simulink model "pn_dopple"  (Simulink 7.2)
settings: Solver=ode45  StartTime=0.0  StopTime=0.02  RelTol=1e-3
libraries: simulink x256, commsynccomp2 x2, dsparch4 x1, commfilt2 x1, commutil2 x1, dspspect3 x1
(part 1 of 3)
settings Model: Creator=Administrator  LastModifiedBy=Administrator
settings OptimizationCC: InitFltsAndDblsToZero=on

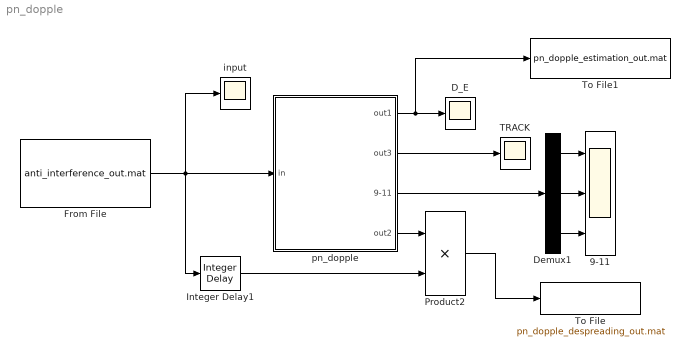
== system pn_dopple ==
  9-11 : Scope  NumInputPorts=3
      settings: YMin=0~0~0  YMax=35~35~40  SaveName=ScopeData3
  D_E : Scope
      settings: TimeRange=0.02  YMin=95  YMax=105  SaveName=ScopeData7
  Demux1 : Demux  Outputs=3
  From File : FromFile  FileName=anti_interference_out.mat  SampleTime=0
  Integer Delay1 : simulink/Discrete/Integer Delay  vinit=0.0  samptime=1/5.1e6  NumDelays=50
  Product2 : Product  OutDataType=sfix(16)  OutScaling=2^0  RndMeth=Zero
  TRACK : Scope
      settings: YMin=-1  YMax=1  SaveName=ScopeData6
  To File : ToFile  Filename=pn_dopple_despreading_out.mat  SampleTime=1/5.1e6
  To File1 : ToFile  Filename=pn_dopple_estimation_out.mat  SampleTime=1/5.1e6
  input : Scope
      settings: YMin=-1  YMax=1  SaveName=ScopeData14
  pn_dopple : Subsystem  TreatAsAtomicUnit=on
  wires:
  pn_dopple/1(out1) -> D_E/1, To File1/1
  pn_dopple/2(out3) -> TRACK/1
  pn_dopple/3(9-11) -> Demux1/1
  Demux1/1 -> 9-11/1
  Demux1/2 -> 9-11/2
  Demux1/3 -> 9-11/3
  From File/1 -> pn_dopple/1(in), Integer Delay1/1, input/1
  pn_dopple/4(out2) -> Product2/1
  Integer Delay1/1 -> Product2/2
  Product2/1 -> To File/1

== system pn_dopple/pn_dopple ==
  in : Inport  OutDataType=sfix(16)  OutScaling=2^0
  "De-Carrier " : Subsystem
  FFT compensate : Subsystem
  Local PN : Subsystem
  MF_Sstem : Subsystem
  Magnitude FFT : dspspect3/Magnitude FFT  SystemSampleTime=-1  mag_or_magsq=Magnitude  fftLenInherit=off  fftsize=32
  MainTain System : Subsystem  TreatAsAtomicUnit=on
  Scope2 : Scope
      settings: TimeRange=0.06427185951473757  YMin=-2  YMax=2  MaxDataPoints=100000
  Sign : Signum
  Zero-Order Hold : ZeroOrderHold  SampleTime=1/255e3
  out1 : Outport  OutDataType=sfix(16)  OutScaling=2^0
  out3 : Outport  Port=2  OutDataType=sfix(16)  OutScaling=2^0
  9-11 : Outport  Port=3  OutDataType=sfix(16)  OutScaling=2^0
  out2 : Outport  Port=4  OutDataType=sfix(16)  OutScaling=2^0
  wires:
  in/1 -> "De-Carrier "/1(in)
  FFT compensate/2(PN Peak) -> Local PN/1(in)
  Zero-Order Hold/1 -> Sign/1
  Sign/1 -> MF_Sstem/1(In1), Local PN/2(in1)
  MF_Sstem/1(bus Out1) -> Magnitude FFT/1
  Magnitude FFT/1 -> FFT compensate/1(In1)
  MainTain System/1(Out1) -> out1/1, Scope2/1
  "De-Carrier "/1(out) -> Zero-Order Hold/1
  Local PN/2(out) -> out3/1
  FFT compensate/3(9-11) -> 9-11/1
  FFT compensate/1(FFT compensate positive) -> MainTain System/Trigger, MainTain System/1(In1)
  Local PN/1(1 0 0 1 1 1 0 1) -> out2/1

== system pn_dopple/pn_dopple/De-Carrier  ==
  note: 5.1e5 Hz
      |
      | 1/5.1e6
      |
      | 255K-300K
  in : Inport  OutDataType=sfix(16)  OutScaling=2^0
  Continuous-Time VCO1 : commsynccomp2/Continuous-Time VCO  SystemSampleTime=-1  Ac=1  Fc=5.0e5  Kc=1000  Ph=pi/2
  Digital Filter Design4 : dsparch4/Digital Filter Design  SystemSampleTime=-1  mwdsp_browser_bugfix_var=off
  Product1 : Product  OutDataType=sfix(16)  OutScaling=2^0  RndMeth=Zero
  Scope1 : Scope
      settings: SaveName=ScopeData4  MaxDataPoints=100000
  Scope3 : Scope
      settings: SaveName=ScopeData16  MaxDataPoints=100000
  Zero-Order Hold1 : ZeroOrderHold  SampleTime=1/5.1e6
  Zero-Order Hold2 : ZeroOrderHold  SampleTime=1/5.1e6
  out : Outport  OutDataType=sfix(16)  OutScaling=2^0
  wires:
  in/1 -> Product1/2
  Product1/1 -> Scope3/1, Zero-Order Hold1/1
  Digital Filter Design4/1 -> out/1, Scope1/1
  Continuous-Time VCO1/1 -> Zero-Order Hold2/1
  Zero-Order Hold2/1 -> Product1/1
  Zero-Order Hold1/1 -> Digital Filter Design4/1

== system pn_dopple/pn_dopple/FFT compensate ==
  In1 : Inport  OutDataType=sfix(16)  OutScaling=2^0
  Demux : Demux  Outputs=32
  Mux : Mux  Inputs=3
  Product1 : Product  OutDataType=sfix(16)  OutScaling=2^0  RndMeth=Zero
  Product8 : Product  OutDataType=sfix(16)  OutScaling=2^0  RndMeth=Zero
  Rate Transition1 : RateTransition  Deterministic=off  OutPortSampleTime=1/5.1e6
  Rate Transition2 : RateTransition  Deterministic=off  OutPortSampleTime=1/5.1e6
  Rate Transition3 : RateTransition  Deterministic=off  OutPortSampleTime=1/5.1e6
  Scope{1..2,4..7} (6 alike) : Scope  NumInputPorts=3
      Scope1 settings: TimeRange=0.06427185951473757  YMin=0~-5~-5  YMax=14~5~5  SaveName=ScopeData9  MaxDataPoints=100000
      Scope2 settings: TimeRange=0.06427185951473757  YMin=0~-5~-5  YMax=14~5~5  SaveName=ScopeData11  MaxDataPoints=100000
      Scope4 settings: TimeRange=0.06427185951473757  YMin=0~-5~-5  YMax=14~5~5  SaveName=ScopeData12  MaxDataPoints=100000
      Scope5 settings: TimeRange=0.06427185951473757  YMin=0~-5~-5  YMax=14~5~5  SaveName=ScopeData13  MaxDataPoints=100000
      Scope6 settings: TimeRange=0.06427185951473757  YMin=0~-5~-5  YMax=14~5~5  SaveName=ScopeData33  MaxDataPoints=100000
      Scope7 settings: TimeRange=0.06427185951473757  YMin=0~-5~-5  YMax=14~5~5  SaveName=ScopeData47  MaxDataPoints=100000
  Scope14 : Scope
      settings: SaveName=ScopeData24  MaxDataPoints=100000
  Scope3 : Scope
      settings: SaveName=ScopeData27  MaxDataPoints=100000
  Step : Step  Time=0.001  SampleTime=0
  Step1 : Step  Time=0.001  SampleTime=0
  Subsystem : Subsystem
  FFT compensate positive : Outport  OutDataType=sfix(16)  OutScaling=2^0
  PN Peak : Outport  Port=2  OutDataType=sfix(16)  OutScaling=2^0
  9-11 : Outport  Port=3  OutDataType=sfix(16)  OutScaling=2^0
  wires:
  Demux/3 -> Subsystem/3(In3), Scope2/3
  Demux/2 -> Subsystem/2(In2), Scope2/2
  Demux/4 -> Scope1/1, Subsystem/4(In4)
  Demux/5 -> Scope1/2, Subsystem/5(In5)
  Demux/6 -> Scope1/3, Subsystem/6(In6)
  Demux/7 -> Subsystem/7(In7), Scope4/1
  Demux/8 -> Subsystem/8(In8), Scope4/2
  Demux/9 -> Subsystem/9(In9), Scope4/3
  Demux/10 -> Subsystem/10(In10), Scope5/1, Mux/1
  Demux/11 -> Subsystem/11(In11), Scope5/2, Mux/2
  Demux/12 -> Subsystem/12(In12), Scope5/3, Mux/3
  Demux/13 -> Subsystem/13(In13), Scope6/1
  Demux/14 -> Subsystem/14(In14), Scope6/2
  Demux/15 -> Subsystem/15(In15), Scope6/3
  In1/1 -> Demux/1
  Demux/1 -> Subsystem/1(In1), Scope2/1
  Subsystem/1(Out1) -> Scope14/1, Product1/1
  Step/1 -> Rate Transition3/1
  Product8/1 -> Rate Transition1/1
  Subsystem/2(Out2) -> Rate Transition2/1
  Rate Transition1/1 -> PN Peak/1, Scope3/1
  Rate Transition2/1 -> Product8/1
  Demux/16 -> Subsystem/16(In16), Scope7/1
  Demux/17 -> Scope7/2
  Demux/18 -> Scope7/3
  Rate Transition3/1 -> Product8/2
  Step1/1 -> Product1/2
  Product1/1 -> FFT compensate positive/1
  Mux/1 -> 9-11/1

== system pn_dopple/pn_dopple/Local PN ==
  in : Inport  OutDataType=sfix(16)  OutScaling=2^0
  in1 : Inport  Port=2  OutDataType=sfix(16)  OutScaling=2^0
  LOCAL_DELAY : Subsystem  TreatAsAtomicUnit=on
  PN_TRACK : Subsystem  TreatAsAtomicUnit=on
  Scope{1..5} (5 alike) : Scope
      Scope1 settings: TimeRange=0.06427185951473757  YMin=-2  YMax=2  SaveName=ScopeData23  MaxDataPoints=100000
      Scope2 settings: TimeRange=0.06427185951473757  YMin=-2  YMax=2  SaveName=ScopeData29  MaxDataPoints=100000
      Scope3 settings: TimeRange=0.06427185951473757  YMin=-2  YMax=2  SaveName=ScopeData18  MaxDataPoints=100000
      Scope4 settings: TimeRange=0.06427185951473757  YMin=-2  YMax=2  SaveName=ScopeData5  MaxDataPoints=100000
      Scope5 settings: TimeRange=0.06427185951473757  YMin=-2  YMax=2  SaveName=ScopeData30  MaxDataPoints=100000
  "local PN " : Subsystem  TreatAsAtomicUnit=on
  logic control : Subsystem  TreatAsAtomicUnit=on
  threshold deside : Subsystem  TreatAsAtomicUnit=on
  threshold deside stop and start : Subsystem
  1 0 0 1 1 1 0 1 : Outport  OutDataType=sfix(16)  OutScaling=2^0
  out : Outport  Port=2  OutDataType=sfix(16)  OutScaling=2^0
  wires:
  logic control/1(Out2) -> Scope5/1, "local PN "/Enable, PN_TRACK/Enable
  threshold deside/1(Out2) -> logic control/1(In1), threshold deside stop and start/1(In1)
  threshold deside stop and start/1(Out1) -> Scope3/1, threshold deside/Enable, Scope4/1
  [A] -> threshold deside stop and start/2(In2)
  in/1 -> threshold deside/1(In1), Scope2/1
  "local PN "/1("1 0 0 1 1 1 0 1 ") -> 1 0 0 1 1 1 0 1/1, Scope1/1, PN_TRACK/1(In1)
  PN_TRACK/1(Out1) -> "local PN "/1(B), out/1
  in1/1 -> LOCAL_DELAY/1(In1)
  LOCAL_DELAY/2(Out1) -> PN_TRACK/3(In3)
  LOCAL_DELAY/1(Out2) -> PN_TRACK/2(In2)

== system pn_dopple/pn_dopple/MF_Sstem ==
  In1 : Inport  OutDataType=sfix(16)  OutScaling=2^0
  Add : Sum  Inputs=++++++++++++++++++++++++++++++++  OutDataType=sfix(16)  OutScaling=2^-10
  MF array : Subsystem
  Mux : Mux  Inputs=32
  Scope14 : Scope
      settings: SaveName=ScopeData34  MaxDataPoints=100000
  Zero-Order Hold : ZeroOrderHold  SampleTime=1/255000
  bus Out1 : Outport  OutDataType=sfix(16)  OutScaling=2^0
  wires:
  In1/1 -> Zero-Order Hold/1
  Zero-Order Hold/1 -> MF array/1(In1)
  Mux/1 -> bus Out1/1
  Add/1 -> Scope14/1
  MF array/1(Out1) -> Mux/1, Add/1
  MF array/2(Out2) -> Mux/2, Add/2
  MF array/3(Out3) -> Mux/3, Add/3
  MF array/4(Out4) -> Mux/4, Add/4
  MF array/5(Out5) -> Mux/5, Add/5
  MF array/6(Out6) -> Mux/6, Add/6
  MF array/7(Out7) -> Mux/7, Add/7
  MF array/8(Out8) -> Mux/8, Add/8
  MF array/9(Out9) -> Mux/9, Add/9
  MF array/10(Out10) -> Mux/10, Add/10
  MF array/11(Out11) -> Mux/11, Add/11
  MF array/12(Out12) -> Mux/12, Add/12
  MF array/13(Out13) -> Mux/13, Add/13
  MF array/14(Out14) -> Mux/14, Add/14
  MF array/15(Out15) -> Mux/15, Add/15
  MF array/16(Out16) -> Mux/16, Add/16
  MF array/17(Out17) -> Mux/17, Add/17
  MF array/18(Out18) -> Mux/18, Add/18
  MF array/19(Out19) -> Mux/19, Add/19
  MF array/20(Out20) -> Mux/20, Add/20
  MF array/21(Out21) -> Mux/21, Add/21
  MF array/22(Out22) -> Mux/22, Add/22
  MF array/23(Out23) -> Mux/23, Add/23
  MF array/24(Out24) -> Mux/24, Add/24
  MF array/25(Out25) -> Mux/25, Add/25
  MF array/26(Out26) -> Mux/26, Add/26
  MF array/27(Out27) -> Mux/27, Add/27
  MF array/28(Out28) -> Mux/28, Add/28
  MF array/29(Out29) -> Mux/29, Add/29
  MF array/30(Out30) -> Mux/30, Add/30
  MF array/31(Out31) -> Mux/31, Add/31
  MF array/32(Out32) -> Mux/32, Add/32

== system pn_dopple/pn_dopple/MainTain System ==
  In1 : Inport  OutDataType=sfix(16)  OutScaling=2^0
  Trigger : TriggerPort
  Out1 : Outport  OutDataType=sfix(16)  OutScaling=2^0
  wires:
  In1/1 -> Out1/1

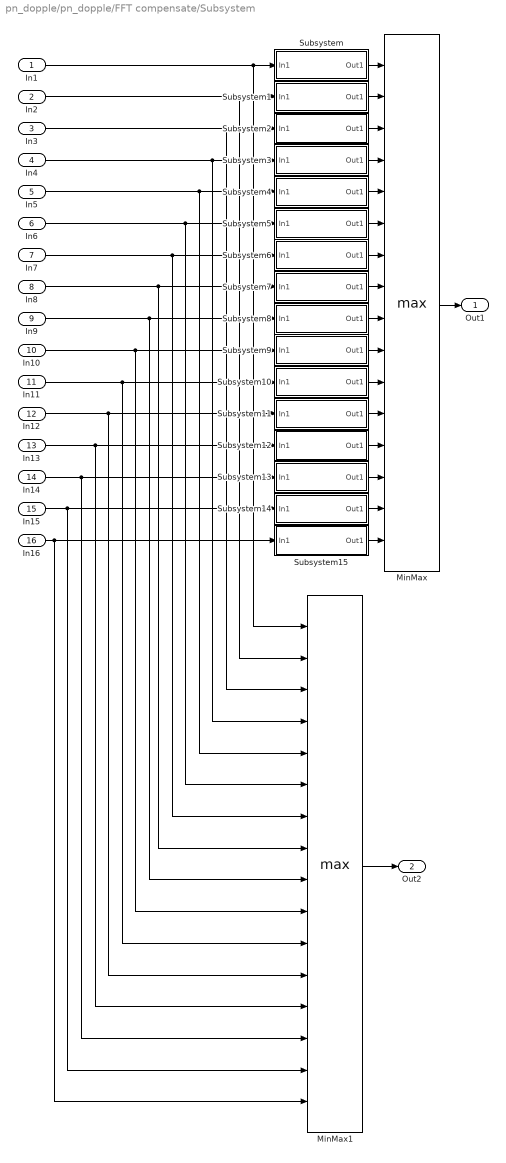
== system pn_dopple/pn_dopple/FFT compensate/Subsystem ==
  In1 : Inport  OutDataType=sfix(16)  OutScaling=2^0
  In2 : Inport  Port=2  OutDataType=sfix(16)  OutScaling=2^0
  In3 : Inport  Port=3  OutDataType=sfix(16)  OutScaling=2^0
  In4 : Inport  Port=4  OutDataType=sfix(16)  OutScaling=2^0
  In5 : Inport  Port=5  OutDataType=sfix(16)  OutScaling=2^0
  In6 : Inport  Port=6  OutDataType=sfix(16)  OutScaling=2^0
  In7 : Inport  Port=7  OutDataType=sfix(16)  OutScaling=2^0
  In8 : Inport  Port=8  OutDataType=sfix(16)  OutScaling=2^0
  In9 : Inport  Port=9  OutDataType=sfix(16)  OutScaling=2^0
  In10 : Inport  Port=10  OutDataType=sfix(16)  OutScaling=2^0
  In11 : Inport  Port=11  OutDataType=sfix(16)  OutScaling=2^0
  In12 : Inport  Port=12  OutDataType=sfix(16)  OutScaling=2^0
  In13 : Inport  Port=13  OutDataType=sfix(16)  OutScaling=2^0
  In14 : Inport  Port=14  OutDataType=sfix(16)  OutScaling=2^0
  In15 : Inport  Port=15  OutDataType=sfix(16)  OutScaling=2^0
  In16 : Inport  Port=16  OutDataType=sfix(16)  OutScaling=2^0
  MinMax : MinMax  Function=max  Inputs=16  OutDataType=sfix(16)  OutScaling=2^0
  MinMax1 : MinMax  Function=max  Inputs=16  OutDataType=sfix(16)  OutScaling=2^0
  Subsystem : Subsystem
  Subsystem1 : Subsystem
  Subsystem10 : Subsystem
  Subsystem11 : Subsystem
  Subsystem12 : Subsystem
  Subsystem13 : Subsystem
  Subsystem14 : Subsystem
  Subsystem15 : Subsystem
  Subsystem2 : Subsystem
  Subsystem3 : Subsystem
  Subsystem4 : Subsystem
  Subsystem5 : Subsystem
  Subsystem6 : Subsystem
  Subsystem7 : Subsystem
  Subsystem8 : Subsystem
  Subsystem9 : Subsystem
  Out1 : Outport  OutDataType=sfix(16)  OutScaling=2^0
  Out2 : Outport  Port=2  OutDataType=sfix(16)  OutScaling=2^0
  wires:
  In1/1 -> Subsystem/1(In1), MinMax1/1
  In2/1 -> Subsystem1/1(In1), MinMax1/2
  In3/1 -> Subsystem2/1(In1), MinMax1/3
  In4/1 -> Subsystem3/1(In1), MinMax1/4
  In5/1 -> Subsystem4/1(In1), MinMax1/5
  In6/1 -> Subsystem5/1(In1), MinMax1/6
  In7/1 -> Subsystem6/1(In1), MinMax1/7
  In8/1 -> Subsystem7/1(In1), MinMax1/8
  In9/1 -> Subsystem8/1(In1), MinMax1/9
  In10/1 -> Subsystem9/1(In1), MinMax1/10
  In11/1 -> Subsystem10/1(In1), MinMax1/11
  In12/1 -> Subsystem11/1(In1), MinMax1/12
  In13/1 -> Subsystem12/1(In1), MinMax1/13
  In14/1 -> Subsystem13/1(In1), MinMax1/14
  In15/1 -> Subsystem14/1(In1), MinMax1/15
  In16/1 -> Subsystem15/1(In1), MinMax1/16
  MinMax/1 -> Out1/1
  Subsystem/1(Out1) -> MinMax/1
  Subsystem1/1(Out1) -> MinMax/2
  Subsystem2/1(Out1) -> MinMax/3
  Subsystem3/1(Out1) -> MinMax/4
  Subsystem4/1(Out1) -> MinMax/5
  Subsystem5/1(Out1) -> MinMax/6
  Subsystem6/1(Out1) -> MinMax/7
  Subsystem7/1(Out1) -> MinMax/8
  Subsystem8/1(Out1) -> MinMax/9
  Subsystem9/1(Out1) -> MinMax/10
  Subsystem10/1(Out1) -> MinMax/11
  Subsystem11/1(Out1) -> MinMax/12
  Subsystem12/1(Out1) -> MinMax/13
  Subsystem13/1(Out1) -> MinMax/14
  Subsystem14/1(Out1) -> MinMax/15
  Subsystem15/1(Out1) -> MinMax/16
  MinMax1/1 -> Out2/1

== system pn_dopple/pn_dopple/Local PN/LOCAL_DELAY ==
  In1 : Inport  OutDataType=sfix(16)  OutScaling=2^0
  Unit Delay : UnitDelay  SampleTime=1/1000000
  Out2 : Outport  OutDataType=sfix(16)  OutScaling=2^0
  Out1 : Outport  Port=2  OutDataType=sfix(16)  OutScaling=2^0
  wires:
  In1/1 -> Unit Delay/1, Out1/1
  Unit Delay/1 -> Out2/1

== system pn_dopple/pn_dopple/Local PN/PN_TRACK ==
  In1 : Inport  OutDataType=sfix(16)  OutScaling=2^0
  In2 : Inport  Port=2  OutDataType=sfix(16)  OutScaling=2^0
  In3 : Inport  Port=3  OutDataType=sfix(16)  OutScaling=2^0
  Enable : EnablePort
  Data Type Conversion : DataTypeConversion  OutDataTypeMode=double  OutDataType=sfix(16)  OutScaling=2^0  OutDataTypeStr=double
  Data Type Conversion1 : DataTypeConversion  OutDataTypeMode=double  OutDataType=sfix(16)  OutScaling=2^0  OutDataTypeStr=double
  Data Type Conversion2 : DataTypeConversion  OutDataTypeMode=double  OutDataType=sfix(16)  OutScaling=2^0  OutDataTypeStr=double
  Gain1 : Gain  Gain=1100/1000  ParameterDataType=sfix(16)  ParameterScaling=2^0  OutDataType=sfix(16)  OutScaling=2^0
  Integrate and Dump : Subsystem
  Memory1 : Memory
  Memory2 : Memory
  Memory3 : Memory
  Product : Product  OutDataType=sfix(16)  OutScaling=2^0  RndMeth=Zero
  Product1 : Product  OutDataType=sfix(16)  OutScaling=2^0  RndMeth=Zero
  Scope : Scope  NumInputPorts=2
      settings: YMin=-5~-5  YMax=5~5  SaveName=ScopeData8
  Sum : Sum  Inputs=-+  OutDataType=sfix(16)  OutScaling=2^0
  Zero-Order Hold : ZeroOrderHold  SampleTime=10
  Zero-Order Hold1 : ZeroOrderHold  SampleTime=10
  Zero-Order Hold2 : ZeroOrderHold  SampleTime=10
  Zero-Order Hold3 : ZeroOrderHold
  Out1 : Outport  OutDataType=sfix(16)  OutScaling=2^0
  wires:
  In1/1 -> Memory1/1
  In2/1 -> Memory2/1
  In3/1 -> Memory3/1
  Data Type Conversion/1 -> Zero-Order Hold/1
  Data Type Conversion1/1 -> Zero-Order Hold1/1
  Data Type Conversion2/1 -> Zero-Order Hold2/1
  Zero-Order Hold/1 -> Product/1, Product1/1
  Zero-Order Hold1/1 -> Product/2
  Zero-Order Hold2/1 -> Product1/2
  Product/1 -> Sum/1, Scope/1
  Product1/1 -> Sum/2, Scope/2
  Sum/1 -> Zero-Order Hold3/1
  Zero-Order Hold3/1 -> Integrate and Dump/1(In1)
  Integrate and Dump/1(Out1) -> Gain1/1
  Memory1/1 -> Data Type Conversion/1
  Memory2/1 -> Data Type Conversion1/1
  Memory3/1 -> Data Type Conversion2/1
  Gain1/1 -> Out1/1

== system pn_dopple/pn_dopple/Local PN/local PN  ==
  B : Inport  OutDataType=sfix(16)  OutScaling=2^0
  Enable : EnablePort  StatesWhenEnabling=reset
  Clock : Subsystem
  Local System : Subsystem
  Scope1 : Scope
      settings: YMin=0.95  YMax=1.05  SaveName=ScopeData10
  Scope2 : Scope
      settings: YMin=0.95  YMax=1.05  SaveName=ScopeData26
  Unipolar to Bipolar Converter : commutil2/Unipolar to Bipolar Converter  SystemSampleTime=-1  M=2  polarity=Positive  dataType=Inherit via internal rule
  "1 0 0 1 1 1 0 1 " : Outport  OutDataType=sfix(16)  OutScaling=2^0
  wires:
  Clock/1(Out1) -> Local System/1(In1), Scope1/1
  Local System/1("[1 0 0 1 1 1 0 1]") -> Unipolar to Bipolar Converter/1
  B/1 -> Clock/1(In2), Scope2/1
  Unipolar to Bipolar Converter/1 -> "1 0 0 1 1 1 0 1 "/1

== system pn_dopple/pn_dopple/Local PN/logic control ==
  In1 : Inport  OutDataType=sfix(16)  OutScaling=2^0
  Triggered Subsystem : Subsystem  TreatAsAtomicUnit=on
  Out2 : Outport  OutDataType=sfix(16)  OutScaling=2^0
  wires:
  Triggered Subsystem/1(Out2) -> Out2/1
  In1/1 -> Triggered Subsystem/Trigger

== system pn_dopple/pn_dopple/Local PN/threshold deside ==
  In1 : Inport  OutDataType=sfix(16)  OutScaling=2^0
  Enable : EnablePort
  Data Type Conversion : DataTypeConversion  OutDataTypeMode=double  OutDataType=sfix(16)  OutScaling=2^0  OutDataTypeStr=double
  Relational Operator : RelationalOperator  Operator=>  LogicOutDataTypeMode=boolean  OutDataTypeStr=boolean
  Scope : Scope
  Scope1 : Scope
      settings: SaveName=ScopeData28
  gate value : Constant  Value=60  OutDataType=sfix(16)  OutScaling=2^0
  Out2 : Outport  OutDataType=sfix(16)  OutScaling=2^0
  wires:
  In1/1 -> Relational Operator/1, Scope1/1
  gate value/1 -> Relational Operator/2
  Relational Operator/1 -> Scope/1, Data Type Conversion/1
  Data Type Conversion/1 -> Out2/1

== system pn_dopple/pn_dopple/Local PN/threshold deside stop and start ==
  In1 : Inport  OutDataType=sfix(16)  OutScaling=2^0
  In2 : Inport  Port=2  OutDataType=sfix(16)  OutScaling=2^0
  Constant : Constant  OutDataType=sfix(16)  OutScaling=2^0
  Logical Operator : Logic  Operator=XOR  AllPortsSameDT=off  OutDataTypeMode=boolean  OutDataTypeStr=boolean
  Logical Operator1 : Logic  Operator=OR  AllPortsSameDT=off  OutDataTypeMode=boolean  OutDataTypeStr=boolean
  Memory1 : Memory  InheritSampleTime=on
  Triggered Subsystem : Subsystem  TreatAsAtomicUnit=on
  Out1 : Outport  OutDataType=sfix(16)  OutScaling=2^0
  wires:
  Triggered Subsystem/1(Out1) -> Logical Operator/2
  Constant/1 -> Logical Operator/1
  Logical Operator/1 -> Memory1/1
  Memory1/1 -> Out1/1
  In1/1 -> Logical Operator1/2
  In2/1 -> Logical Operator1/1
  Logical Operator1/1 -> Triggered Subsystem/Trigger

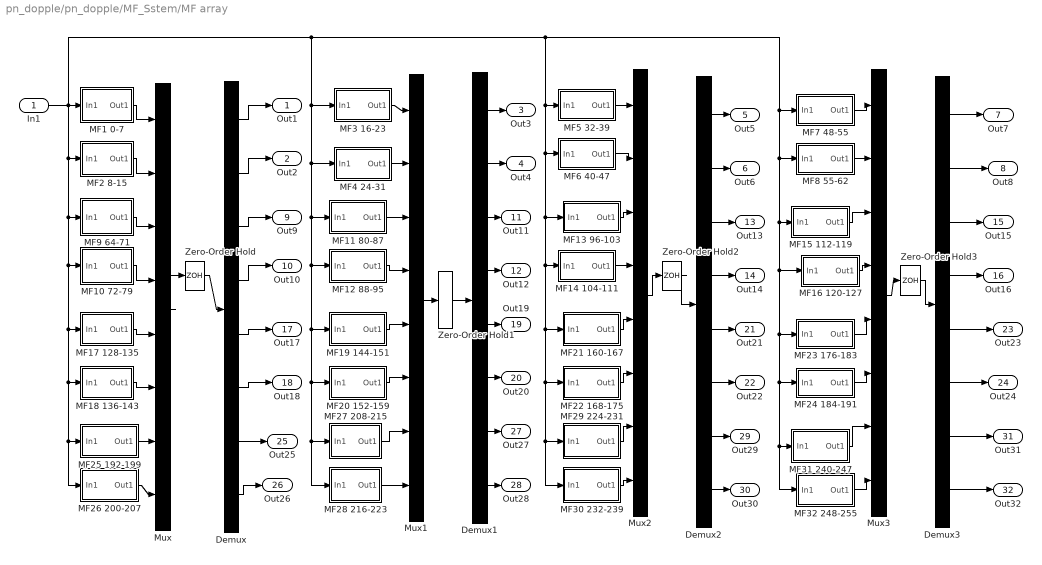
== system pn_dopple/pn_dopple/MF_Sstem/MF array ==
  In1 : Inport  OutDataType=sfix(16)  OutScaling=2^0
  Demux{,1..3} (4 alike) : Demux  Outputs=8
  MF1 0-7 : Subsystem
  MF10 72-79 : Subsystem
  MF11 80-87 : Subsystem
  MF12 88-95 : Subsystem
  MF13 96-103 : Subsystem
  MF14 104-111 : Subsystem
  MF15 112-119 : Subsystem
  MF16 120-127 : Subsystem
  MF17 128-135 : Subsystem
  MF18 136-143 : Subsystem
  MF19 144-151 : Subsystem
  MF2 8-15 : Subsystem
  MF20 152-159 : Subsystem
  MF21 160-167 : Subsystem
  MF22 168-175 : Subsystem
  MF23 176-183 : Subsystem
  MF24 184-191 : Subsystem
  MF25 192-199 : Subsystem
  MF26 200-207 : Subsystem
  MF27 208-215 : Subsystem
  MF28 216-223 : Subsystem
  MF29 224-231 : Subsystem
  MF3 16-23 : Subsystem
  MF30 232-239 : Subsystem
  MF31 240-247 : Subsystem
  MF32 248-255 : Subsystem
  MF4 24-31 : Subsystem
  MF5 32-39 : Subsystem
  MF6 40-47 : Subsystem
  MF7 48-55 : Subsystem
  MF8 55-62 : Subsystem
  MF9 64-71 : Subsystem
  Mux{,1..3} (4 alike) : Mux  Inputs=8
  Zero-Order Hold{,1..3} (4 alike) : ZeroOrderHold  SampleTime=1/255000
  Out1 : Outport  OutDataType=sfix(16)  OutScaling=2^0
  Out2 : Outport  Port=2  OutDataType=sfix(16)  OutScaling=2^0
  Out3 : Outport  Port=3  OutDataType=sfix(16)  OutScaling=2^0
  Out4 : Outport  Port=4  OutDataType=sfix(16)  OutScaling=2^0
  Out5 : Outport  Port=5  OutDataType=sfix(16)  OutScaling=2^0
  Out6 : Outport  Port=6  OutDataType=sfix(16)  OutScaling=2^0
  Out7 : Outport  Port=7  OutDataType=sfix(16)  OutScaling=2^0
  Out8 : Outport  Port=8  OutDataType=sfix(16)  OutScaling=2^0
  Out9 : Outport  Port=9  OutDataType=sfix(16)  OutScaling=2^0
  Out10 : Outport  Port=10  OutDataType=sfix(16)  OutScaling=2^0
  Out11 : Outport  Port=11  OutDataType=sfix(16)  OutScaling=2^0
  Out12 : Outport  Port=12  OutDataType=sfix(16)  OutScaling=2^0
  Out13 : Outport  Port=13  OutDataType=sfix(16)  OutScaling=2^0
  Out14 : Outport  Port=14  OutDataType=sfix(16)  OutScaling=2^0
  Out15 : Outport  Port=15  OutDataType=sfix(16)  OutScaling=2^0
  Out16 : Outport  Port=16  OutDataType=sfix(16)  OutScaling=2^0
  Out17 : Outport  Port=17  OutDataType=sfix(16)  OutScaling=2^0
  Out18 : Outport  Port=18  OutDataType=sfix(16)  OutScaling=2^0
  Out19 : Outport  Port=19  OutDataType=sfix(16)  OutScaling=2^0
  Out20 : Outport  Port=20  OutDataType=sfix(16)  OutScaling=2^0
  Out21 : Outport  Port=21  OutDataType=sfix(16)  OutScaling=2^0
  Out22 : Outport  Port=22  OutDataType=sfix(16)  OutScaling=2^0
  Out23 : Outport  Port=23  OutDataType=sfix(16)  OutScaling=2^0
  Out24 : Outport  Port=24  OutDataType=sfix(16)  OutScaling=2^0
  Out25 : Outport  Port=25  OutDataType=sfix(16)  OutScaling=2^0
  Out26 : Outport  Port=26  OutDataType=sfix(16)  OutScaling=2^0
  Out27 : Outport  Port=27  OutDataType=sfix(16)  OutScaling=2^0
  Out28 : Outport  Port=28  OutDataType=sfix(16)  OutScaling=2^0
  Out29 : Outport  Port=29  OutDataType=sfix(16)  OutScaling=2^0
  Out30 : Outport  Port=30  OutDataType=sfix(16)  OutScaling=2^0
  Out31 : Outport  Port=31  OutDataType=sfix(16)  OutScaling=2^0
  Out32 : Outport  Port=32  OutDataType=sfix(16)  OutScaling=2^0
  wires:
  Zero-Order Hold3/1 -> Demux3/1
  Mux3/1 -> Zero-Order Hold3/1
  Zero-Order Hold2/1 -> Demux2/1
  Mux2/1 -> Zero-Order Hold2/1
  Zero-Order Hold1/1 -> Demux1/1
  Mux1/1 -> Zero-Order Hold1/1
  Zero-Order Hold/1 -> Demux/1
  Mux/1 -> Zero-Order Hold/1
  In1/1 -> MF1 0-7/1(In1), MF3 16-23/1(In1), MF11 80-87/1(In1), MF19 144-151/1(In1), MF20 152-159/1(In1), MF27 208-215/1(In1), MF28 216-223/1(In1), MF12 88-95/1(In1), MF4 24-31/1(In1), MF5 32-39/1(In1), MF13 96-103/1(In1), MF21 160-167/1(In1), MF22 168-175/1(In1), MF29 224-231/1(In1), MF30 232-239/1(In1), MF14 104-111/1(In1), MF6 40-47/1(In1), MF7 48-55/1(In1), MF23 176-183/1(In1), MF24 184-191/1(In1), MF31 240-247/1(In1), MF32 248-255/1(In1), MF16 120-127/1(In1), MF15 112-119/1(In1), MF8 55-62/1(In1), MF9 64-71/1(In1), MF17 128-135/1(In1), MF18 136-143/1(In1), MF25 192-199/1(In1), MF26 200-207/1(In1), MF10 72-79/1(In1), MF2 8-15/1(In1)
  MF1 0-7/1(Out1) -> Mux/1
  MF2 8-15/1(Out1) -> Mux/2
  MF9 64-71/1(Out1) -> Mux/3
  MF10 72-79/1(Out1) -> Mux/4
  MF17 128-135/1(Out1) -> Mux/5
  MF18 136-143/1(Out1) -> Mux/6
  MF25 192-199/1(Out1) -> Mux/7
  MF26 200-207/1(Out1) -> Mux/8
  Demux/1 -> Out1/1
  Demux/2 -> Out2/1
  Demux/3 -> Out9/1
  Demux/4 -> Out10/1
  Demux/5 -> Out17/1
  Demux/6 -> Out18/1
  Demux/7 -> Out25/1
  Demux/8 -> Out26/1
  MF3 16-23/1(Out1) -> Mux1/1
  MF4 24-31/1(Out1) -> Mux1/2
  MF11 80-87/1(Out1) -> Mux1/3
  MF12 88-95/1(Out1) -> Mux1/4
  MF19 144-151/1(Out1) -> Mux1/5
  MF20 152-159/1(Out1) -> Mux1/6
  MF27 208-215/1(Out1) -> Mux1/7
  MF28 216-223/1(Out1) -> Mux1/8
  Demux1/1 -> Out3/1
  Demux1/2 -> Out4/1
  Demux1/3 -> Out11/1
  Demux1/4 -> Out12/1
  Demux1/5 -> Out19/1
  Demux1/6 -> Out20/1
  Demux1/7 -> Out27/1
  Demux1/8 -> Out28/1
  MF5 32-39/1(Out1) -> Mux2/1
  MF6 40-47/1(Out1) -> Mux2/2
  MF13 96-103/1(Out1) -> Mux2/3
  MF14 104-111/1(Out1) -> Mux2/4
  MF21 160-167/1(Out1) -> Mux2/5
  MF22 168-175/1(Out1) -> Mux2/6
  MF29 224-231/1(Out1) -> Mux2/7
  MF30 232-239/1(Out1) -> Mux2/8
  Demux2/1 -> Out5/1
  Demux2/2 -> Out6/1
  Demux2/3 -> Out13/1
  Demux2/4 -> Out14/1
  Demux2/5 -> Out21/1
  Demux2/6 -> Out22/1
  Demux2/7 -> Out29/1
  Demux2/8 -> Out30/1
  MF7 48-55/1(Out1) -> Mux3/1
  MF8 55-62/1(Out1) -> Mux3/2
  MF15 112-119/1(Out1) -> Mux3/3
  MF16 120-127/1(Out1) -> Mux3/4
  MF23 176-183/1(Out1) -> Mux3/5
  MF24 184-191/1(Out1) -> Mux3/6
  MF31 240-247/1(Out1) -> Mux3/7
  MF32 248-255/1(Out1) -> Mux3/8
  Demux3/1 -> Out7/1
  Demux3/2 -> Out8/1
  Demux3/3 -> Out15/1
  Demux3/4 -> Out16/1
  Demux3/5 -> Out23/1
  Demux3/6 -> Out24/1
  Demux3/7 -> Out31/1
  Demux3/8 -> Out32/1

== system pn_dopple/pn_dopple/FFT compensate/Subsystem/Subsystem ==
  In1 : Inport  OutDataType=sfix(16)  OutScaling=2^0
  Constant : Constant  OutDataType=sfix(16)  OutScaling=2^0
  Constant1 : Constant  Value=0  OutDataType=sfix(16)  OutScaling=2^0
  Constant2 : Constant  Value=0  OutDataType=sfix(16)  OutScaling=2^0
  Product : Product  OutDataType=sfix(16)  OutScaling=2^0  RndMeth=Zero
  Switch : Switch  Threshold=65
  Out1 : Outport  OutDataType=sfix(16)  OutScaling=2^0
  wires:
  Constant/1 -> Switch/1
  Constant1/1 -> Switch/3
  Switch/1 -> Product/1
  Constant2/1 -> Product/2
  In1/1 -> Switch/2
  Product/1 -> Out1/1

== system pn_dopple/pn_dopple/FFT compensate/Subsystem/Subsystem1 ==
  In1 : Inport  OutDataType=sfix(16)  OutScaling=2^0
  Constant : Constant  OutDataType=sfix(16)  OutScaling=2^0
  Constant1 : Constant  Value=0  OutDataType=sfix(16)  OutScaling=2^0
  Constant2 : Constant  Value=10  OutDataType=sfix(16)  OutScaling=2^0
  Product : Product  OutDataType=sfix(16)  OutScaling=2^0  RndMeth=Zero
  Switch : Switch  Threshold=65
  Out1 : Outport  OutDataType=sfix(16)  OutScaling=2^0
  wires:
  Product/1 -> Out1/1
  In1/1 -> Switch/2
  Constant2/1 -> Product/2
  Switch/1 -> Product/1
  Constant1/1 -> Switch/3
  Constant/1 -> Switch/1

== system pn_dopple/pn_dopple/FFT compensate/Subsystem/Subsystem10 ==
  In1 : Inport  OutDataType=sfix(16)  OutScaling=2^0
  Constant : Constant  OutDataType=sfix(16)  OutScaling=2^0
  Constant1 : Constant  Value=0  OutDataType=sfix(16)  OutScaling=2^0
  Constant2 : Constant  Value=100  OutDataType=sfix(16)  OutScaling=2^0
  Product : Product  OutDataType=sfix(16)  OutScaling=2^0  RndMeth=Zero
  Switch : Switch  Threshold=65
  Out1 : Outport  OutDataType=sfix(16)  OutScaling=2^0
  wires:
  Constant/1 -> Switch/1
  Constant1/1 -> Switch/3
  Switch/1 -> Product/1
  Constant2/1 -> Product/2
  In1/1 -> Switch/2
  Product/1 -> Out1/1

== system pn_dopple/pn_dopple/FFT compensate/Subsystem/Subsystem11 ==
  In1 : Inport  OutDataType=sfix(16)  OutScaling=2^0
  Constant : Constant  OutDataType=sfix(16)  OutScaling=2^0
  Constant1 : Constant  Value=0  OutDataType=sfix(16)  OutScaling=2^0
  Constant2 : Constant  Value=110  OutDataType=sfix(16)  OutScaling=2^0
  Product : Product  OutDataType=sfix(16)  OutScaling=2^0  RndMeth=Zero
  Switch : Switch  Threshold=65
  Out1 : Outport  OutDataType=sfix(16)  OutScaling=2^0
  wires:
  Product/1 -> Out1/1
  In1/1 -> Switch/2
  Constant2/1 -> Product/2
  Switch/1 -> Product/1
  Constant1/1 -> Switch/3
  Constant/1 -> Switch/1

== system pn_dopple/pn_dopple/FFT compensate/Subsystem/Subsystem12 ==
  In1 : Inport  OutDataType=sfix(16)  OutScaling=2^0
  Constant : Constant  OutDataType=sfix(16)  OutScaling=2^0
  Constant1 : Constant  Value=0  OutDataType=sfix(16)  OutScaling=2^0
  Constant2 : Constant  Value=120  OutDataType=sfix(16)  OutScaling=2^0
  Product : Product  OutDataType=sfix(16)  OutScaling=2^0  RndMeth=Zero
  Switch : Switch  Threshold=65
  Out1 : Outport  OutDataType=sfix(16)  OutScaling=2^0
  wires:
  Constant/1 -> Switch/1
  Constant1/1 -> Switch/3
  Switch/1 -> Product/1
  Constant2/1 -> Product/2
  In1/1 -> Switch/2
  Product/1 -> Out1/1

== system pn_dopple/pn_dopple/FFT compensate/Subsystem/Subsystem13 ==
  In1 : Inport  OutDataType=sfix(16)  OutScaling=2^0
  Constant : Constant  OutDataType=sfix(16)  OutScaling=2^0
  Constant1 : Constant  Value=0  OutDataType=sfix(16)  OutScaling=2^0
  Constant2 : Constant  Value=130  OutDataType=sfix(16)  OutScaling=2^0
  Product : Product  OutDataType=sfix(16)  OutScaling=2^0  RndMeth=Zero
  Switch : Switch  Threshold=65
  Out1 : Outport  OutDataType=sfix(16)  OutScaling=2^0
  wires:
  Product/1 -> Out1/1
  In1/1 -> Switch/2
  Constant2/1 -> Product/2
  Switch/1 -> Product/1
  Constant1/1 -> Switch/3
  Constant/1 -> Switch/1

== system pn_dopple/pn_dopple/FFT compensate/Subsystem/Subsystem14 ==
  In1 : Inport  OutDataType=sfix(16)  OutScaling=2^0
  Constant : Constant  OutDataType=sfix(16)  OutScaling=2^0
  Constant1 : Constant  Value=0  OutDataType=sfix(16)  OutScaling=2^0
  Constant2 : Constant  Value=140  OutDataType=sfix(16)  OutScaling=2^0
  Product : Product  OutDataType=sfix(16)  OutScaling=2^0  RndMeth=Zero
  Switch : Switch  Threshold=65
  Out1 : Outport  OutDataType=sfix(16)  OutScaling=2^0
  wires:
  Constant/1 -> Switch/1
  Constant1/1 -> Switch/3
  Switch/1 -> Product/1
  Constant2/1 -> Product/2
  In1/1 -> Switch/2
  Product/1 -> Out1/1

== system pn_dopple/pn_dopple/FFT compensate/Subsystem/Subsystem15 ==
  In1 : Inport  OutDataType=sfix(16)  OutScaling=2^0
  Constant : Constant  OutDataType=sfix(16)  OutScaling=2^0
  Constant1 : Constant  Value=0  OutDataType=sfix(16)  OutScaling=2^0
  Constant2 : Constant  Value=150  OutDataType=sfix(16)  OutScaling=2^0
  Product : Product  OutDataType=sfix(16)  OutScaling=2^0  RndMeth=Zero
  Switch : Switch  Threshold=65
  Out1 : Outport  OutDataType=sfix(16)  OutScaling=2^0
  wires:
  Product/1 -> Out1/1
  In1/1 -> Switch/2
  Constant2/1 -> Product/2
  Switch/1 -> Product/1
  Constant1/1 -> Switch/3
  Constant/1 -> Switch/1

== system pn_dopple/pn_dopple/FFT compensate/Subsystem/Subsystem2 ==
  In1 : Inport  OutDataType=sfix(16)  OutScaling=2^0
  Constant : Constant  OutDataType=sfix(16)  OutScaling=2^0
  Constant1 : Constant  Value=0  OutDataType=sfix(16)  OutScaling=2^0
  Constant2 : Constant  Value=20  OutDataType=sfix(16)  OutScaling=2^0
  Product : Product  OutDataType=sfix(16)  OutScaling=2^0  RndMeth=Zero
  Switch : Switch  Threshold=65
  Out1 : Outport  OutDataType=sfix(16)  OutScaling=2^0
  wires:
  Constant/1 -> Switch/1
  Constant1/1 -> Switch/3
  Switch/1 -> Product/1
  Constant2/1 -> Product/2
  In1/1 -> Switch/2
  Product/1 -> Out1/1

== system pn_dopple/pn_dopple/FFT compensate/Subsystem/Subsystem3 ==
  In1 : Inport  OutDataType=sfix(16)  OutScaling=2^0
  Constant : Constant  OutDataType=sfix(16)  OutScaling=2^0
  Constant1 : Constant  Value=0  OutDataType=sfix(16)  OutScaling=2^0
  Constant2 : Constant  Value=30  OutDataType=sfix(16)  OutScaling=2^0
  Product : Product  OutDataType=sfix(16)  OutScaling=2^0  RndMeth=Zero
  Switch : Switch  Threshold=65
  Out1 : Outport  OutDataType=sfix(16)  OutScaling=2^0
  wires:
  Product/1 -> Out1/1
  In1/1 -> Switch/2
  Constant2/1 -> Product/2
  Switch/1 -> Product/1
  Constant1/1 -> Switch/3
  Constant/1 -> Switch/1

== system pn_dopple/pn_dopple/FFT compensate/Subsystem/Subsystem4 ==
  In1 : Inport  OutDataType=sfix(16)  OutScaling=2^0
  Constant : Constant  OutDataType=sfix(16)  OutScaling=2^0
  Constant1 : Constant  Value=0  OutDataType=sfix(16)  OutScaling=2^0
  Constant2 : Constant  Value=40  OutDataType=sfix(16)  OutScaling=2^0
  Product : Product  OutDataType=sfix(16)  OutScaling=2^0  RndMeth=Zero
  Switch : Switch  Threshold=65
  Out1 : Outport  OutDataType=sfix(16)  OutScaling=2^0
  wires:
  Constant/1 -> Switch/1
  Constant1/1 -> Switch/3
  Switch/1 -> Product/1
  Constant2/1 -> Product/2
  In1/1 -> Switch/2
  Product/1 -> Out1/1

== system pn_dopple/pn_dopple/FFT compensate/Subsystem/Subsystem5 ==
  In1 : Inport  OutDataType=sfix(16)  OutScaling=2^0
  Constant : Constant  OutDataType=sfix(16)  OutScaling=2^0
  Constant1 : Constant  Value=0  OutDataType=sfix(16)  OutScaling=2^0
  Constant2 : Constant  Value=50  OutDataType=sfix(16)  OutScaling=2^0
  Product : Product  OutDataType=sfix(16)  OutScaling=2^0  RndMeth=Zero
  Switch : Switch  Threshold=65
  Out1 : Outport  OutDataType=sfix(16)  OutScaling=2^0
  wires:
  Product/1 -> Out1/1
  In1/1 -> Switch/2
  Constant2/1 -> Product/2
  Switch/1 -> Product/1
  Constant1/1 -> Switch/3
  Constant/1 -> Switch/1

== system pn_dopple/pn_dopple/FFT compensate/Subsystem/Subsystem6 ==
  In1 : Inport  OutDataType=sfix(16)  OutScaling=2^0
  Constant : Constant  OutDataType=sfix(16)  OutScaling=2^0
  Constant1 : Constant  Value=0  OutDataType=sfix(16)  OutScaling=2^0
  Constant2 : Constant  Value=60  OutDataType=sfix(16)  OutScaling=2^0
  Product : Product  OutDataType=sfix(16)  OutScaling=2^0  RndMeth=Zero
  Switch : Switch  Threshold=65
  Out1 : Outport  OutDataType=sfix(16)  OutScaling=2^0
  wires:
  Constant/1 -> Switch/1
  Constant1/1 -> Switch/3
  Switch/1 -> Product/1
  Constant2/1 -> Product/2
  In1/1 -> Switch/2
  Product/1 -> Out1/1

== system pn_dopple/pn_dopple/FFT compensate/Subsystem/Subsystem7 ==
  In1 : Inport  OutDataType=sfix(16)  OutScaling=2^0
  Constant : Constant  OutDataType=sfix(16)  OutScaling=2^0
  Constant1 : Constant  Value=0  OutDataType=sfix(16)  OutScaling=2^0
  Constant2 : Constant  Value=70  OutDataType=sfix(16)  OutScaling=2^0
  Product : Product  OutDataType=sfix(16)  OutScaling=2^0  RndMeth=Zero
  Switch : Switch  Threshold=65
  Out1 : Outport  OutDataType=sfix(16)  OutScaling=2^0
  wires:
  Product/1 -> Out1/1
  In1/1 -> Switch/2
  Constant2/1 -> Product/2
  Switch/1 -> Product/1
  Constant1/1 -> Switch/3
  Constant/1 -> Switch/1

== system pn_dopple/pn_dopple/FFT compensate/Subsystem/Subsystem8 ==
  In1 : Inport  OutDataType=sfix(16)  OutScaling=2^0
  Constant : Constant  OutDataType=sfix(16)  OutScaling=2^0
  Constant1 : Constant  Value=0  OutDataType=sfix(16)  OutScaling=2^0
  Constant2 : Constant  Value=80  OutDataType=sfix(16)  OutScaling=2^0
  Product : Product  OutDataType=sfix(16)  OutScaling=2^0  RndMeth=Zero
  Switch : Switch  Threshold=65
  Out1 : Outport  OutDataType=sfix(16)  OutScaling=2^0
  wires:
  Constant/1 -> Switch/1
  Constant1/1 -> Switch/3
  Switch/1 -> Product/1
  Constant2/1 -> Product/2
  In1/1 -> Switch/2
  Product/1 -> Out1/1

== system pn_dopple/pn_dopple/FFT compensate/Subsystem/Subsystem9 ==
  In1 : Inport  OutDataType=sfix(16)  OutScaling=2^0
  Constant : Constant  OutDataType=sfix(16)  OutScaling=2^0
  Constant1 : Constant  Value=0  OutDataType=sfix(16)  OutScaling=2^0
  Constant2 : Constant  Value=90  OutDataType=sfix(16)  OutScaling=2^0
  Product : Product  OutDataType=sfix(16)  OutScaling=2^0  RndMeth=Zero
  Switch : Switch  Threshold=65
  Out1 : Outport  OutDataType=sfix(16)  OutScaling=2^0
  wires:
  Product/1 -> Out1/1
  In1/1 -> Switch/2
  Constant2/1 -> Product/2
  Switch/1 -> Product/1
  Constant1/1 -> Switch/3
  Constant/1 -> Switch/1

== system pn_dopple/pn_dopple/Local PN/PN_TRACK/Integrate and Dump ==
  In1 : Inport
  Gain : Gain  Gain=1/1000  ParameterDataType=sfix(16)  ParameterScaling=2^0  OutDataType=sfix(16)  OutScaling=2^0
  Integrate and Dump : commfilt2/Integrate and Dump  DialogController=commDDGCreate  DialogControllerArgs=DataTag1  obssamples=8  offsetsamples=0  nodump=off  roundingMode=Floor  overflowMode=off
  Memory : Memory  InheritSampleTime=on
  Step : Step  Time=0.0055  SampleTime=0
  Step1 : Step  Time=0.005  SampleTime=0
  Sum1 : Sum  Inputs=-+  OutDataType=sfix(16)  OutScaling=2^0
  Sum2 : Sum  OutDataType=sfix(16)  OutScaling=2^0
  Out1 : Outport
  wires:
  Integrate and Dump/1 -> Gain/1
  Step1/1 -> Sum1/2
  Step/1 -> Sum1/1
  Gain/1 -> Sum2/1
  Sum1/1 -> Sum2/2
  Sum2/1 -> Memory/1
  In1/1 -> Integrate and Dump/1
  Memory/1 -> Out1/1

== system pn_dopple/pn_dopple/Local PN/local PN /Clock ==
  In2 : Inport  Orientation=left  OutDataType=sfix(16)  OutScaling=2^0
  Constant : Constant  Orientation=left  OutDataType=sfix(16)  OutScaling=2^0
  Constant1 : Constant  Orientation=left  Value=0  OutDataType=sfix(16)  OutScaling=2^0
  Continuous-Time VCO : commsynccomp2/Continuous-Time VCO  Orientation=left  SystemSampleTime=-1  Ac=1  Fc=255000  Kc=0.15  Ph=-pi/2
  Switch : Switch  Orientation=left
  Zero-Order Hold : ZeroOrderHold  Orientation=left  SampleTime=1000
  Out1 : Outport  Orientation=left  OutDataType=sfix(16)  OutScaling=2^0
  wires:
  Constant1/1 -> Switch/3
  Constant/1 -> Switch/1
  Continuous-Time VCO/1 -> Switch/2
  Switch/1 -> Out1/1
  In2/1 -> Zero-Order Hold/1
  Zero-Order Hold/1 -> Continuous-Time VCO/1

== system pn_dopple/pn_dopple/Local PN/local PN /Local System ==
  In1 : Inport  OutDataType=sfix(16)  OutScaling=2^0
  Data Type Conversion : DataTypeConversion  OutDataTypeMode=double  OutDataType=sfix(16)  OutScaling=2^0  OutDataTypeStr=double
  Zero-Order Hold3 : ZeroOrderHold  SampleTime=1/255e3
  "[1 0 0 1 1 1 0 1]PN" : Subsystem  TreatAsAtomicUnit=on
  "[1 0 0 1 1 1 0 1]" : Outport  OutDataType=sfix(16)  OutScaling=2^0
  wires:
  In1/1 -> "[1 0 0 1 1 1 0 1]PN"/Trigger, "[1 0 0 1 1 1 0 1]PN"/1(In1)
  "[1 0 0 1 1 1 0 1]PN"/1(Out1) -> Data Type Conversion/1
  Zero-Order Hold3/1 -> "[1 0 0 1 1 1 0 1]"/1
  Data Type Conversion/1 -> Zero-Order Hold3/1

== system pn_dopple/pn_dopple/Local PN/logic control/Triggered Subsystem ==
  Trigger : TriggerPort
  Constant : Constant  OutDataType=sfix(16)  OutScaling=2^0
  Logical Operator : Logic  Operator=XOR  AllPortsSameDT=off  OutDataTypeMode=boolean  OutDataTypeStr=boolean
  Scope : Scope
      settings: SaveName=ScopeData2
  Unit Delay : UnitDelay  Orientation=left  SampleTime=-1
  Out2 : Outport  OutDataType=sfix(16)  OutScaling=2^0
  wires:
  Constant/1 -> Logical Operator/1
  Logical Operator/1 -> Scope/1, Out2/1, Unit Delay/1
  Unit Delay/1 -> Logical Operator/2

== system pn_dopple/pn_dopple/Local PN/threshold deside stop and start/Triggered Subsystem ==
  Trigger : TriggerPort
  Constant1 : Constant  OutDataType=sfix(16)  OutScaling=2^0
  Logical Operator : Logic  Operator=XOR  AllPortsSameDT=off  OutDataTypeMode=boolean  OutDataTypeStr=boolean
  Unit Delay : UnitDelay  Orientation=left  SampleTime=-1
  Out1 : Outport  OutDataType=sfix(16)  OutScaling=2^0
  wires:
  Unit Delay/1 -> Logical Operator/2
  Logical Operator/1 -> Out1/1, Unit Delay/1
  Constant1/1 -> Logical Operator/1

== system pn_dopple/pn_dopple/MF_Sstem/MF array/MF1 0-7 ==
  In1 : Inport  OutDataType=sfix(16)  OutScaling=2^0
  Add : Sum  Inputs=++++++++  OutDataType=sfix(16)  OutScaling=2^-10
  Subsystem : Subsystem
  Out1 : Outport  OutDataType=sfix(16)  OutScaling=2^0
  wires:
  Add/1 -> Out1/1
  In1/1 -> Subsystem/1(In1)
  Subsystem/1(Out1) -> Add/1
  Subsystem/2(Out2) -> Add/2
  Subsystem/3(Out3) -> Add/3
  Subsystem/4(Out4) -> Add/4
  Subsystem/5(Out5) -> Add/5
  Subsystem/6(Out6) -> Add/6
  Subsystem/7(Out7) -> Add/7
  Subsystem/8(Out8) -> Add/8

== system pn_dopple/pn_dopple/MF_Sstem/MF array/MF10 72-79 ==
  In1 : Inport  OutDataType=sfix(16)  OutScaling=2^0
  Add : Sum  Inputs=++++++++  OutDataType=sfix(16)  OutScaling=2^-10
  Subsystem : Subsystem
  Out1 : Outport  OutDataType=sfix(16)  OutScaling=2^0
  wires:
  Subsystem/8(Out8) -> Add/8
  Subsystem/7(Out7) -> Add/7
  Subsystem/6(Out6) -> Add/6
  Subsystem/5(Out5) -> Add/5
  Subsystem/4(Out4) -> Add/4
  Subsystem/3(Out3) -> Add/3
  Subsystem/2(Out2) -> Add/2
  Subsystem/1(Out1) -> Add/1
  In1/1 -> Subsystem/1(In1)
  Add/1 -> Out1/1

== system pn_dopple/pn_dopple/MF_Sstem/MF array/MF11 80-87 ==
  In1 : Inport  OutDataType=sfix(16)  OutScaling=2^0
  Add : Sum  Inputs=++++++++  OutDataType=sfix(16)  OutScaling=2^-10
  Subsystem : Subsystem
  Out1 : Outport  OutDataType=sfix(16)  OutScaling=2^0
  wires:
  In1/1 -> Subsystem/1(In1)
  Add/1 -> Out1/1
  Subsystem/1(Out3) -> Add/1
  Subsystem/2(Out4) -> Add/2
  Subsystem/3(Out7) -> Add/3
  Subsystem/4(Out8) -> Add/4
  Subsystem/5(Out9) -> Add/5
  Subsystem/6(Out11) -> Add/6
  Subsystem/7(Out14) -> Add/7
  Subsystem/8(Out15) -> Add/8

== system pn_dopple/pn_dopple/MF_Sstem/MF array/MF12 88-95 ==
  In1 : Inport  OutDataType=sfix(16)  OutScaling=2^0
  Add : Sum  Inputs=++++++++  OutDataType=sfix(16)  OutScaling=2^-10
  Subsystem : Subsystem
  Out1 : Outport  OutDataType=sfix(16)  OutScaling=2^0
  wires:
  Add/1 -> Out1/1
  In1/1 -> Subsystem/1(In1)
  Subsystem/1(Out1) -> Add/1
  Subsystem/2(Out5) -> Add/2
  Subsystem/3(Out10) -> Add/3
  Subsystem/4(Out12) -> Add/4
  Subsystem/5(Out13) -> Add/5
  Subsystem/6(Out16) -> Add/6
  Subsystem/7(Out17) -> Add/7
  Subsystem/8(Out18) -> Add/8

== system pn_dopple/pn_dopple/MF_Sstem/MF array/MF13 96-103 ==
  In1 : Inport  OutDataType=sfix(16)  OutScaling=2^0
  Add : Sum  Inputs=++++++++  OutDataType=sfix(16)  OutScaling=2^-10
  Subsystem : Subsystem
  Out1 : Outport  OutDataType=sfix(16)  OutScaling=2^0
  wires:
  Add/1 -> Out1/1
  In1/1 -> Subsystem/1(In1)
  Subsystem/1(Out3) -> Add/1
  Subsystem/2(Out4) -> Add/2
  Subsystem/3(Out7) -> Add/3
  Subsystem/4(Out8) -> Add/4
  Subsystem/5(Out9) -> Add/5
  Subsystem/6(Out11) -> Add/6
  Subsystem/7(Out14) -> Add/7
  Subsystem/8(Out15) -> Add/8

== system pn_dopple/pn_dopple/MF_Sstem/MF array/MF14 104-111 ==
  In1 : Inport  OutDataType=sfix(16)  OutScaling=2^0
  Add : Sum  Inputs=++++++++  OutDataType=sfix(16)  OutScaling=2^-10
  Subsystem : Subsystem
  Out1 : Outport  OutDataType=sfix(16)  OutScaling=2^0
  wires:
  In1/1 -> Subsystem/1(In1)
  Add/1 -> Out1/1
  Subsystem/1(Out1) -> Add/1
  Subsystem/2(Out5) -> Add/2
  Subsystem/3(Out10) -> Add/3
  Subsystem/4(Out12) -> Add/4
  Subsystem/5(Out13) -> Add/5
  Subsystem/6(Out16) -> Add/6
  Subsystem/7(Out17) -> Add/7
  Subsystem/8(Out18) -> Add/8

== system pn_dopple/pn_dopple/MF_Sstem/MF array/MF15 112-119 ==
  In1 : Inport  OutDataType=sfix(16)  OutScaling=2^0
  Add : Sum  Inputs=++++++++  OutDataType=sfix(16)  OutScaling=2^-10
  Subsystem : Subsystem
  Out1 : Outport  OutDataType=sfix(16)  OutScaling=2^0
  wires:
  In1/1 -> Subsystem/1(In1)
  Add/1 -> Out1/1
  Subsystem/1(Out3) -> Add/1
  Subsystem/2(Out4) -> Add/2
  Subsystem/3(Out7) -> Add/3
  Subsystem/4(Out8) -> Add/4
  Subsystem/5(Out9) -> Add/5
  Subsystem/6(Out11) -> Add/6
  Subsystem/7(Out14) -> Add/7
  Subsystem/8(Out15) -> Add/8

== system pn_dopple/pn_dopple/MF_Sstem/MF array/MF16 120-127 ==
  In1 : Inport  OutDataType=sfix(16)  OutScaling=2^0
  Add : Sum  Inputs=++++++++  OutDataType=sfix(16)  OutScaling=2^-10
  Subsystem : Subsystem
  Out1 : Outport  OutDataType=sfix(16)  OutScaling=2^0
  wires:
  Add/1 -> Out1/1
  In1/1 -> Subsystem/1(In1)
  Subsystem/1(Out1) -> Add/1
  Subsystem/2(Out5) -> Add/2
  Subsystem/3(Out10) -> Add/3
  Subsystem/4(Out12) -> Add/4
  Subsystem/5(Out13) -> Add/5
  Subsystem/6(Out16) -> Add/6
  Subsystem/7(Out17) -> Add/7
  Subsystem/8(Out18) -> Add/8

== system pn_dopple/pn_dopple/MF_Sstem/MF array/MF17 128-135 ==
  In1 : Inport  OutDataType=sfix(16)  OutScaling=2^0
  Add : Sum  Inputs=++++++++  OutDataType=sfix(16)  OutScaling=2^-10
  Subsystem : Subsystem
  Out1 : Outport  OutDataType=sfix(16)  OutScaling=2^0
  wires:
  In1/1 -> Subsystem/1(In1)
  Add/1 -> Out1/1
  Subsystem/1(Out3) -> Add/1
  Subsystem/2(Out4) -> Add/2
  Subsystem/3(Out7) -> Add/3
  Subsystem/4(Out8) -> Add/4
  Subsystem/5(Out9) -> Add/5
  Subsystem/6(Out11) -> Add/6
  Subsystem/7(Out14) -> Add/7
  Subsystem/8(Out15) -> Add/8

== system pn_dopple/pn_dopple/MF_Sstem/MF array/MF18 136-143 ==
  In1 : Inport  OutDataType=sfix(16)  OutScaling=2^0
  Add : Sum  Inputs=++++++++  OutDataType=sfix(16)  OutScaling=2^-10
  Subsystem : Subsystem
  Out1 : Outport  OutDataType=sfix(16)  OutScaling=2^0
  wires:
  Add/1 -> Out1/1
  In1/1 -> Subsystem/1(In1)
  Subsystem/1(Out1) -> Add/1
  Subsystem/2(Out5) -> Add/2
  Subsystem/3(Out10) -> Add/3
  Subsystem/4(Out12) -> Add/4
  Subsystem/5(Out13) -> Add/5
  Subsystem/6(Out16) -> Add/6
  Subsystem/7(Out17) -> Add/7
  Subsystem/8(Out18) -> Add/8

== system pn_dopple/pn_dopple/MF_Sstem/MF array/MF19 144-151 ==
  In1 : Inport  OutDataType=sfix(16)  OutScaling=2^0
  Add : Sum  Inputs=++++++++  OutDataType=sfix(16)  OutScaling=2^-10
  Subsystem : Subsystem
  Out1 : Outport  OutDataType=sfix(16)  OutScaling=2^0
  wires:
  Add/1 -> Out1/1
  In1/1 -> Subsystem/1(In1)
  Subsystem/1(Out3) -> Add/1
  Subsystem/2(Out4) -> Add/2
  Subsystem/3(Out7) -> Add/3
  Subsystem/4(Out8) -> Add/4
  Subsystem/5(Out9) -> Add/5
  Subsystem/6(Out11) -> Add/6
  Subsystem/7(Out14) -> Add/7
  Subsystem/8(Out15) -> Add/8

== system pn_dopple/pn_dopple/MF_Sstem/MF array/MF2 8-15 ==
  In1 : Inport  OutDataType=sfix(16)  OutScaling=2^0
  Add : Sum  Inputs=++++++++  OutDataType=sfix(16)  OutScaling=2^-10
  Subsystem : Subsystem
  Out1 : Outport  OutDataType=sfix(16)  OutScaling=2^0
  wires:
  Subsystem/8(Out8) -> Add/8
  Subsystem/7(Out7) -> Add/7
  Subsystem/6(Out6) -> Add/6
  Subsystem/5(Out5) -> Add/5
  Subsystem/4(Out4) -> Add/4
  Subsystem/3(Out3) -> Add/3
  Subsystem/2(Out2) -> Add/2
  Subsystem/1(Out1) -> Add/1
  In1/1 -> Subsystem/1(In1)
  Add/1 -> Out1/1

== system pn_dopple/pn_dopple/MF_Sstem/MF array/MF20 152-159 ==
  In1 : Inport  OutDataType=sfix(16)  OutScaling=2^0
  Add : Sum  Inputs=++++++++  OutDataType=sfix(16)  OutScaling=2^-10
  Subsystem : Subsystem
  Out1 : Outport  OutDataType=sfix(16)  OutScaling=2^0
  wires:
  In1/1 -> Subsystem/1(In1)
  Add/1 -> Out1/1
  Subsystem/1(Out1) -> Add/1
  Subsystem/2(Out5) -> Add/2
  Subsystem/3(Out10) -> Add/3
  Subsystem/4(Out12) -> Add/4
  Subsystem/5(Out13) -> Add/5
  Subsystem/6(Out16) -> Add/6
  Subsystem/7(Out17) -> Add/7
  Subsystem/8(Out18) -> Add/8

== system pn_dopple/pn_dopple/MF_Sstem/MF array/MF21 160-167 ==
  In1 : Inport  OutDataType=sfix(16)  OutScaling=2^0
  Add : Sum  Inputs=++++++++  OutDataType=sfix(16)  OutScaling=2^-10
  Subsystem : Subsystem
  Out1 : Outport  OutDataType=sfix(16)  OutScaling=2^0
  wires:
  In1/1 -> Subsystem/1(In1)
  Add/1 -> Out1/1
  Subsystem/1(Out3) -> Add/1
  Subsystem/2(Out4) -> Add/2
  Subsystem/3(Out7) -> Add/3
  Subsystem/4(Out8) -> Add/4
  Subsystem/5(Out9) -> Add/5
  Subsystem/6(Out11) -> Add/6
  Subsystem/7(Out14) -> Add/7
  Subsystem/8(Out15) -> Add/8

== system pn_dopple/pn_dopple/MF_Sstem/MF array/MF22 168-175 ==
  In1 : Inport  OutDataType=sfix(16)  OutScaling=2^0
  Add : Sum  Inputs=++++++++  OutDataType=sfix(16)  OutScaling=2^-10
  Subsystem : Subsystem
  Out1 : Outport  OutDataType=sfix(16)  OutScaling=2^0
  wires:
  Add/1 -> Out1/1
  In1/1 -> Subsystem/1(In1)
  Subsystem/1(Out1) -> Add/1
  Subsystem/2(Out5) -> Add/2
  Subsystem/3(Out10) -> Add/3
  Subsystem/4(Out12) -> Add/4
  Subsystem/5(Out13) -> Add/5
  Subsystem/6(Out16) -> Add/6
  Subsystem/7(Out17) -> Add/7
  Subsystem/8(Out18) -> Add/8

== system pn_dopple/pn_dopple/MF_Sstem/MF array/MF23 176-183 ==
  In1 : Inport  OutDataType=sfix(16)  OutScaling=2^0
  Add : Sum  Inputs=++++++++  OutDataType=sfix(16)  OutScaling=2^-10
  Subsystem : Subsystem
  Out1 : Outport  OutDataType=sfix(16)  OutScaling=2^0
  wires:
  Add/1 -> Out1/1
  In1/1 -> Subsystem/1(In1)
  Subsystem/1(Out3) -> Add/1
  Subsystem/2(Out4) -> Add/2
  Subsystem/3(Out7) -> Add/3
  Subsystem/4(Out8) -> Add/4
  Subsystem/5(Out9) -> Add/5
  Subsystem/6(Out11) -> Add/6
  Subsystem/7(Out14) -> Add/7
  Subsystem/8(Out15) -> Add/8

== system pn_dopple/pn_dopple/MF_Sstem/MF array/MF24 184-191 ==
  In1 : Inport  OutDataType=sfix(16)  OutScaling=2^0
  Add : Sum  Inputs=++++++++  OutDataType=sfix(16)  OutScaling=2^-10
  Subsystem : Subsystem
  Out1 : Outport  OutDataType=sfix(16)  OutScaling=2^0
  wires:
  In1/1 -> Subsystem/1(In1)
  Add/1 -> Out1/1
  Subsystem/1(Out1) -> Add/1
  Subsystem/2(Out5) -> Add/2
  Subsystem/3(Out10) -> Add/3
  Subsystem/4(Out12) -> Add/4
  Subsystem/5(Out13) -> Add/5
  Subsystem/6(Out16) -> Add/6
  Subsystem/7(Out17) -> Add/7
  Subsystem/8(Out18) -> Add/8

== system pn_dopple/pn_dopple/MF_Sstem/MF array/MF25 192-199 ==
  In1 : Inport  OutDataType=sfix(16)  OutScaling=2^0
  Add : Sum  Inputs=++++++++  OutDataType=sfix(16)  OutScaling=2^-10
  Subsystem : Subsystem
  Out1 : Outport  OutDataType=sfix(16)  OutScaling=2^0
  wires:
  In1/1 -> Subsystem/1(In1)
  Add/1 -> Out1/1
  Subsystem/1(Out3) -> Add/1
  Subsystem/2(Out4) -> Add/2
  Subsystem/3(Out7) -> Add/3
  Subsystem/4(Out8) -> Add/4
  Subsystem/5(Out9) -> Add/5
  Subsystem/6(Out11) -> Add/6
  Subsystem/7(Out14) -> Add/7
  Subsystem/8(Out15) -> Add/8

== system pn_dopple/pn_dopple/MF_Sstem/MF array/MF26 200-207 ==
  In1 : Inport  OutDataType=sfix(16)  OutScaling=2^0
  Add : Sum  Inputs=++++++++  OutDataType=sfix(16)  OutScaling=2^-10
  Subsystem : Subsystem
  Out1 : Outport  OutDataType=sfix(16)  OutScaling=2^0
  wires:
  Add/1 -> Out1/1
  In1/1 -> Subsystem/1(In1)
  Subsystem/1(Out1) -> Add/1
  Subsystem/2(Out5) -> Add/2
  Subsystem/3(Out10) -> Add/3
  Subsystem/4(Out12) -> Add/4
  Subsystem/5(Out13) -> Add/5
  Subsystem/6(Out16) -> Add/6
  Subsystem/7(Out17) -> Add/7
  Subsystem/8(Out18) -> Add/8

== system pn_dopple/pn_dopple/MF_Sstem/MF array/MF27 208-215 ==
  In1 : Inport  OutDataType=sfix(16)  OutScaling=2^0
  Add : Sum  Inputs=++++++++  OutDataType=sfix(16)  OutScaling=2^-10
  Subsystem : Subsystem
  Out1 : Outport  OutDataType=sfix(16)  OutScaling=2^0
  wires:
  Add/1 -> Out1/1
  In1/1 -> Subsystem/1(In1)
  Subsystem/1(Out3) -> Add/1
  Subsystem/2(Out4) -> Add/2
  Subsystem/3(Out7) -> Add/3
  Subsystem/4(Out8) -> Add/4
  Subsystem/5(Out9) -> Add/5
  Subsystem/6(Out11) -> Add/6
  Subsystem/7(Out14) -> Add/7
  Subsystem/8(Out15) -> Add/8

== system pn_dopple/pn_dopple/MF_Sstem/MF array/MF28 216-223 ==
  In1 : Inport  OutDataType=sfix(16)  OutScaling=2^0
  Add : Sum  Inputs=++++++++  OutDataType=sfix(16)  OutScaling=2^-10
  Subsystem : Subsystem
  Out1 : Outport  OutDataType=sfix(16)  OutScaling=2^0
  wires:
  In1/1 -> Subsystem/1(In1)
  Add/1 -> Out1/1
  Subsystem/1(Out1) -> Add/1
  Subsystem/2(Out5) -> Add/2
  Subsystem/3(Out10) -> Add/3
  Subsystem/4(Out12) -> Add/4
  Subsystem/5(Out13) -> Add/5
  Subsystem/6(Out16) -> Add/6
  Subsystem/7(Out17) -> Add/7
  Subsystem/8(Out18) -> Add/8
